simulink model "Vrs_calc"  (Simulink 8.9)
settings: Solver=ode45  StartTime=0.0  StopTime=10.0  RelTol=1e-3  EnableMultiTasking=on
settings Model: SuppressorTable=22 serialization::archive 11 0 6 0 0 0 0 0  Creator=hlopez5  LastModifiedBy=judithlopez
settings DataIOCC: SignalLoggingSaveFormat=Dataset
settings DebuggingCC: UnderspecifiedInitializationDetection=Simplified  MergeDetectMultiDrivingBlocksExec=error  SolverPrmCheckMsg=warning  FcnCallInpInsideContextMsg=error
settings GRTTargetCC: CombineOutputUpdateFcns=on  GRTInterface=off

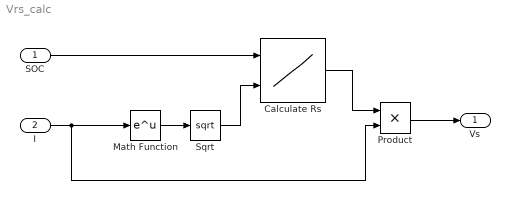
== system Vrs_calc ==
  SOC : Inport
  I : Inport  Port=2
  Calculate Rs : Lookup_n-D  BreakpointsForDimension1=[1,2,3]  BreakpointsForDimension2=[1,2,3]  Table=reshape([6,0,0.0083,9,0.70845,0.005,18,1.2391,0.0027],3,3)  RndMeth=Simplest  InputSameDT=on
  Math Function : Math  SaturateOnIntegerOverflow=on
  Product : Product
  Sqrt : Sqrt  SaturateOnIntegerOverflow=on
  Vs : Outport
  wires:
  I/1 -> Product/2, Math Function/1
  Math Function/1 -> Sqrt/1
  Sqrt/1 -> Calculate Rs/2
  SOC/1 -> Calculate Rs/1
  Calculate Rs/1 -> Product/1
  Product/1 -> Vs/1
